simulink model "battery_logic"  (R2019b)
settings: Solver=VariableStepAuto  StartTime=0.0  StopTime=600  MaxStep=1  RelTol=1e-3
values from neighbouring files (symbols this model uses):
  I_BC_max = -input (4)    [battchargedischarge.m]    (also in demoEPS.m = 3; demoEPS_R2019a.m = 3; demoEPS_v1.m = 3; demoEPS_v1a.m = 3)
  I_BD_max = input (3)    [battchargedischarge.m]    (also in demoEPS.m = 5; demoEPS_R2019a.m = 5; demoEPS_v1.m = 5; demoEPS_v1a.m = 5)
  iB = 2    [testsim.m]
libraries: simulink x1
settings Model: Creator=Ricardo  LastModifiedBy=Ricardo

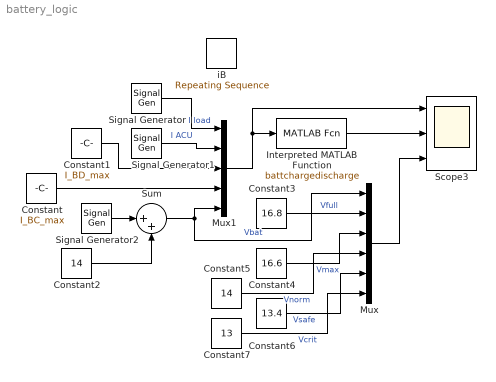
== system battery_logic ==
  Constant : Constant  Value=I_BC_max
  Constant1 : Constant  Value=I_BD_max
  Constant2 : Constant  Value=14
  Constant3 : Constant  Value=16.8
  Constant4 : Constant  Value=16.6
  Constant5 : Constant  Value=14
  Constant6 : Constant  Value=13.4
  Constant7 : Constant  Value=13
  Interpreted MATLAB Function : MATLABFcn  MATLABFcn=battchargedischarge
  Mux : Mux  Inputs=6
  Mux1 : Mux  Inputs=5
  Scope3 : Scope  NumInputPorts=3
  Signal Generator : SignalGenerator  WaveForm=sawtooth  Amplitude=3*iB  Frequency=0.5/300
  Signal Generator1 : SignalGenerator  Amplitude=3*iB  Frequency=0.5/300
  Signal Generator2 : SignalGenerator  Amplitude=3  Frequency=0.05  Units=rad/sec
  Sum : Sum  Inputs=|++
  iB : simulink/Sources/Repeating Sequence  rep_seq_t=[0 200 205 300 305]  rep_seq_y=[iB iB -iB -iB iB]
  wires:
  Interpreted MATLAB Function/1 -> Scope3/2
  Mux1/1 -> Scope3/1, Interpreted MATLAB Function/1
  Constant1/1 -> Mux1/3
  Signal Generator1/1 -> Mux1/2  "I ACU"
  Constant/1 -> Mux1/4
  Signal Generator/1 -> Mux1/1  "I load"
  Signal Generator2/1 -> Sum/1
  Constant2/1 -> Sum/2
  Sum/1 -> Mux/1, Mux1/5  "Vbat"
  Mux/1 -> Scope3/3
  Constant3/1 -> Mux/2  "Vfull"
  Constant4/1 -> Mux/3  "Vmax"
  Constant5/1 -> Mux/4  "Vnorm"
  Constant6/1 -> Mux/5  "Vsafe"
  Constant7/1 -> Mux/6  "Vcrit"
